simulink model "bitwise_operator"  (R2021a)
settings: Solver=VariableStepAuto  StartTime=0.0  StopTime=10.0  RelTol=1e-3
libraries: simulink x5
settings Model: Creator=lenovo  LastModifiedBy=lenovo

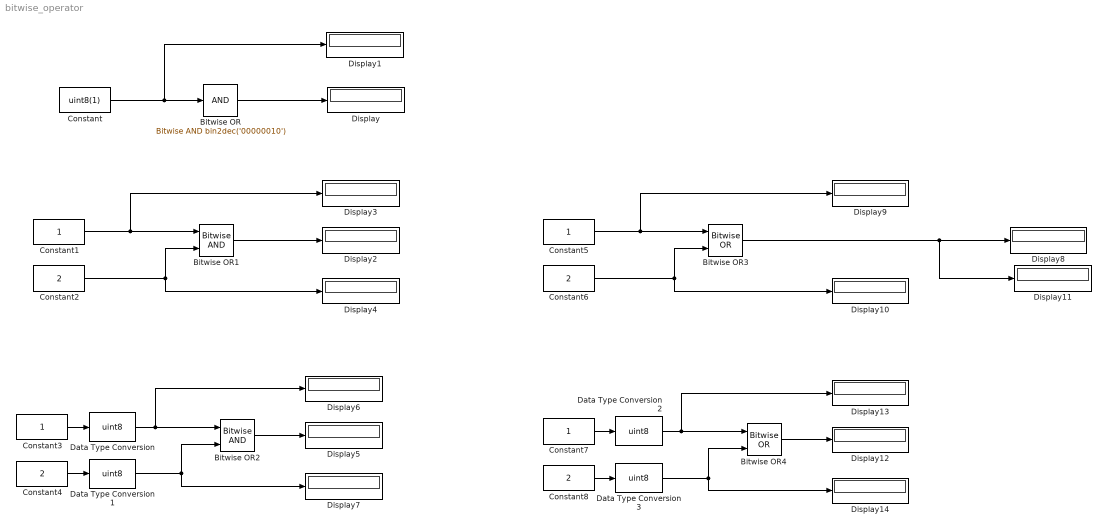
== system bitwise_operator ==
  Bitwise OR : simulink/Logic and Bit Operations/Bitwise Operator  logicop=AND  UseBitMask=on  BitMask=bin2dec('00000010')  BitMaskRealWorld=Stored Integer
  Bitwise OR1 : simulink/Logic and Bit Operations/Bitwise Operator  logicop=AND  UseBitMask=off  NumInputPorts=2  BitMask=bin2dec('00000010')  BitMaskRealWorld=Stored Integer
  Bitwise OR2 : simulink/Logic and Bit Operations/Bitwise Operator  logicop=AND  UseBitMask=off  NumInputPorts=2  BitMask=bin2dec('00000010')  BitMaskRealWorld=Stored Integer
  Bitwise OR3 : simulink/Logic and Bit Operations/Bitwise Operator  logicop=OR  UseBitMask=off  NumInputPorts=2  BitMask=bin2dec('00000010')  BitMaskRealWorld=Stored Integer
  Bitwise OR4 : simulink/Logic and Bit Operations/Bitwise Operator  logicop=OR  UseBitMask=off  NumInputPorts=2  BitMask=bin2dec('00000010')  BitMaskRealWorld=Stored Integer
  Constant : Constant  Value=uint8(1)
  Constant1 : Constant  OutDataTypeStr=uint8
  Constant2 : Constant  Value=2  OutDataTypeStr=uint8
  Constant3 : Constant
  Constant4 : Constant  Value=2
  Constant5 : Constant  OutDataTypeStr=uint8
  Constant6 : Constant  Value=2  OutDataTypeStr=uint8
  Constant7 : Constant
  Constant8 : Constant  Value=2
  Data Type Conversion{,1..3} (4 alike) : DataTypeConversion  OutDataTypeStr=uint8
  Display{,1..14} (15 alike) : Display
      Display settings: Format=binary (Stored Integer)
      Display1 settings: Format=binary (Stored Integer)
      Display10 settings: Format=binary (Stored Integer)
      Display12 settings: Format=binary (Stored Integer)
      Display13 settings: Format=binary (Stored Integer)
      Display14 settings: Format=binary (Stored Integer)
      Display2 settings: Format=binary (Stored Integer)
      Display3 settings: Format=binary (Stored Integer)
      Display4 settings: Format=binary (Stored Integer)
      Display5 settings: Format=binary (Stored Integer)
      Display6 settings: Format=binary (Stored Integer)
      Display7 settings: Format=binary (Stored Integer)
      Display8 settings: Format=binary (Stored Integer)
      Display9 settings: Format=binary (Stored Integer)
  wires:
  Constant/1 -> Display1/1, Bitwise OR/1
  Bitwise OR/1 -> Display/1
  Constant1/1 -> Display3/1, Bitwise OR1/1
  Constant2/1 -> Display4/1, Bitwise OR1/2
  Bitwise OR1/1 -> Display2/1
  Bitwise OR2/1 -> Display5/1
  Constant4/1 -> Data Type Conversion1/1
  Constant3/1 -> Data Type Conversion/1
  Data Type Conversion/1 -> Bitwise OR2/1, Display6/1
  Data Type Conversion1/1 -> Bitwise OR2/2, Display7/1
  Bitwise OR3/1 -> Display11/1, Display8/1
  Constant6/1 -> Bitwise OR3/2, Display10/1
  Constant5/1 -> Bitwise OR3/1, Display9/1
  Data Type Conversion3/1 -> Display14/1, Bitwise OR4/2
  Data Type Conversion2/1 -> Display13/1, Bitwise OR4/1
  Constant7/1 -> Data Type Conversion2/1
  Constant8/1 -> Data Type Conversion3/1
  Bitwise OR4/1 -> Display12/1
